simulink model "math_2_test"  (Simulink 8.4)
settings: Solver=VariableStepDiscrete  StartTime=0.0  StopTime=10.0  RelTol=1e-3
settings Model: Creator=arnaud  LastModifiedBy=arnaud
settings DataIOCC: SaveFormat=Structure

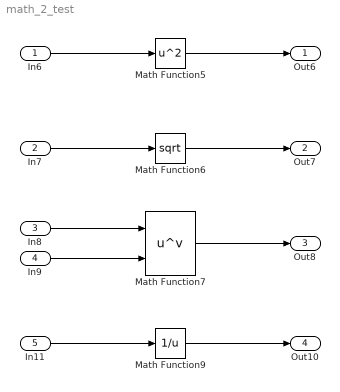
== system math_2_test ==
  In6 : Inport
  In7 : Inport  Port=2
  In8 : Inport  Port=3
  In9 : Inport  Port=4
  In11 : Inport  Port=5
  Math Function5 : Math  Operator=square  SaturateOnIntegerOverflow=on
  Math Function6 : Math  Operator=sqrt  SaturateOnIntegerOverflow=on
  Math Function7 : Math  Operator=pow  SaturateOnIntegerOverflow=on
  Math Function9 : Math  Operator=reciprocal  SaturateOnIntegerOverflow=on
  Out6 : Outport
  Out7 : Outport  Port=2
  Out8 : Outport  Port=3
  Out10 : Outport  Port=4
  wires:
  In6/1 -> Math Function5/1
  Math Function5/1 -> Out6/1
  In7/1 -> Math Function6/1
  Math Function6/1 -> Out7/1
  In8/1 -> Math Function7/1
  In9/1 -> Math Function7/2
  Math Function7/1 -> Out8/1
  In11/1 -> Math Function9/1
  Math Function9/1 -> Out10/1
